simulink model "FO_PLL"  (R2025b)
settings: Solver=VariableStepAuto  StartTime=0.0  StopTime=10.0  RelTol=1e-3
values from neighbouring files (symbols this model uses):
  a0 = alpha^alpha + 2.*alpha + 1    (= 2.70710678119)    [Fractional_order_Filter.m]
  a1 = (a2 - a0) .* tan((2 + alpha) .* pi./4)    [Fractional_order_Filter.m]
  a2 = alpha^alpha - 2.*alpha + 1    (= 0.707106781187)    [Fractional_order_Filter.m]
  SNR_dB = 20    [Fractional_order_Filter.m]
  zeta = tan(alpha*pi/2)+sec(alpha*pi/2)    [Fractional_order_Filter.m]    (also in Fractional_order_Filter_orderd.m)
libraries: simulink x1
settings Model: Creator=amahd  LastModifiedBy=amahd

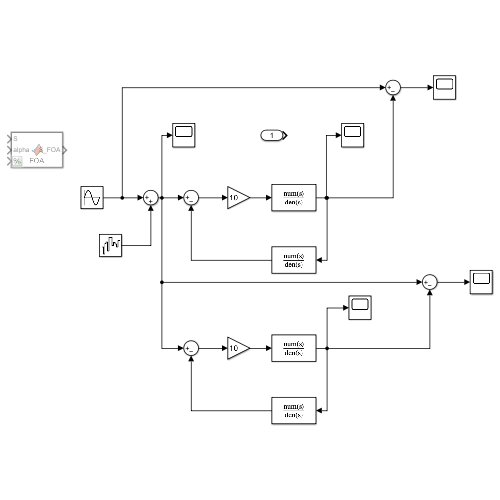
[thumbnail: Simulink's stored preview of the top-level diagram]
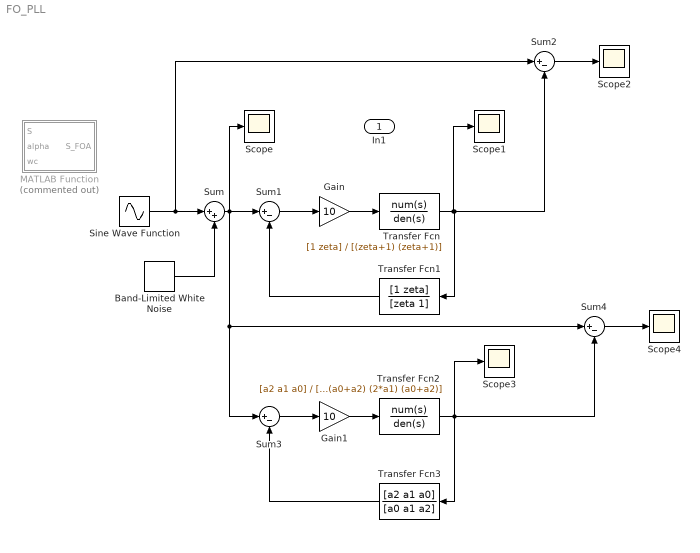
== system FO_PLL ==
  In1 : Inport
  Band-Limited White Noise : simulink/Sources/Band-Limited White Noise  Cov=[0.5/(10^(SNR_dB/10))]  Ts=0.1  seed=[23341]
  Gain : Gain  Gain=10
  Gain1 : Gain  Gain=10
  MATLAB Function : MATLAB Function  Commented=on  TreatAsAtomicUnit=on
  Scope{,1..4} (5 alike) : Scope
      Scope settings: ActiveDisplayYMinimum=-4.3659816079745832  ActiveDisplayYMaximum=3.2138170170450873
      Scope1 settings: ActiveDisplayYMinimum=-4.3659816079745832  ActiveDisplayYMaximum=3.2138170170450873
      Scope2 settings: ActiveDisplayYMinimum=-4.3659816079745832  ActiveDisplayYMaximum=3.2138170170450873  DataLoggingVariableName=ScopeData2
      Scope3 settings: ActiveDisplayYMinimum=-4.3659816079745832  ActiveDisplayYMaximum=3.2138170170450873  DataLoggingVariableName=ScopeData3
      Scope4 settings: ActiveDisplayYMinimum=-4.3659816079745832  ActiveDisplayYMaximum=3.2138170170450873  DataLoggingVariableName=ScopeData4
  Sine Wave Function : Sin  Frequency=2*pi*10  SampleTime=0
  Sum : Sum  Inputs=|++
  Sum{1..4} (4 alike) : Sum  Inputs=|+-
  Transfer Fcn : TransferFcn  Numerator=[1 zeta]  Denominator=[(zeta+1) (zeta+1)]
  Transfer Fcn1 : TransferFcn  Numerator=[1 zeta]  Denominator=[zeta 1]
  Transfer Fcn2 : TransferFcn  Numerator=[a2 a1 a0]  Denominator=[(a0+a2) (2*a1) (a0+a2)]
  Transfer Fcn3 : TransferFcn  Numerator=[a2 a1 a0]  Denominator=[a0 a1 a2]
  wires:
  Sine Wave Function/1 -> Sum2/1, Sum/1
  Sum/1 -> Sum4/1, Sum3/1, Sum1/1, Scope/1
  Band-Limited White Noise/1 -> Sum/2
  Gain/1 -> Transfer Fcn/1
  Sum1/1 -> Gain/1
  Transfer Fcn/1 -> Sum2/2, Transfer Fcn1/1, Scope1/1
  Transfer Fcn1/1 -> Sum1/2
  Sum2/1 -> Scope2/1
  Transfer Fcn3/1 -> Sum3/2
  Transfer Fcn2/1 -> Sum4/2, Transfer Fcn3/1, Scope3/1
  Gain1/1 -> Transfer Fcn2/1
  Sum3/1 -> Gain1/1
  Sum4/1 -> Scope4/1

== matlab function FO_PLL/MATLAB Function ==
  data: S input; S_FOA output; alpha input; wc input
function S_FOA = FOA(S, alpha, wc)
    Zeta=tan(alpha*pi/2)+sec(alpha*pi/2);
    S_FOA = (S .* Zeta ./ wc + 1) ./ (S ./ wc + Zeta) ;
end
